simulink model "Rebuild"  (R2024b)
settings: Solver=VariableStepAuto  StartTime=0.0  StopTime=12  RelTol=1e-3
values from neighbouring files (symbols this model uses):
  A = 1.1    [RT14e_Parameters.m]    (also in RT15e_Parameters.m = 1.088; RT15evo_Parameters.m = 1.088)
  Aero_balance = 55    [RT14e_Parameters.m]    (also in RT15e_Parameters.m; RT15evo_Parameters.m)
  Aeromaps_ON = 0    [SIM_setup.m]
  air_density = 1.2    [SIM_setup.m]
  Balance_FW = Data_FW_STD(1:end,2)    [RT15e_Parameters.m]    (also in RT15evo_Parameters.m)
  Balance_R_11 = Data_R_11(1:end,2)    [RT15e_Parameters.m]    (also in RT15evo_Parameters.m)
  Br_coef_of_friction_F = 0.33    [RT14e_Parameters.m]    (also in RT15e_Parameters.m; RT15evo_Parameters.m)
  Br_coef_of_friction_R = 0.33    [RT14e_Parameters.m]    (also in RT15e_Parameters.m; RT15evo_Parameters.m)
  Br_pistons_area_F = 3617.26/1e6    (= 0.00361726)    [RT14e_Parameters.m]    (also in RT15e_Parameters.m; RT15evo_Parameters.m)
  Br_pistons_area_R = 2026.83/1e6    (= 0.00202683)    [RT14e_Parameters.m]    (also in RT15e_Parameters.m; RT15evo_Parameters.m)
  CdA = 1.31*A    (= 1.441)    [RT14e_Parameters.m]    (also in RT15e_Parameters.m = 1.700544; RT15evo_Parameters.m = 1.700544)
  CdA_FW = Data_FW_STD(1:end,3)    [RT15e_Parameters.m]    (also in RT15evo_Parameters.m)
  CdA_R_11 = Data_R_11(1:end,3)    [RT15e_Parameters.m]    (also in RT15evo_Parameters.m)
  ClA = 3.3*A    (= 3.63)    [RT14e_Parameters.m]    (also in RT15e_Parameters.m = 4.36288; RT15evo_Parameters.m = 4.36288)
  ClA_FW = Data_FW_STD(1:end,4)    [RT15e_Parameters.m]    (also in RT15evo_Parameters.m)
  ClA_R_11 = Data_R_11(1:end,4)    [RT15e_Parameters.m]    (also in RT15evo_Parameters.m)
  CoG_z = 0.35    [RT14e_Parameters.m]    (also in RT15e_Parameters.m = 0.28495; RT15evo_Parameters.m = 0.28495)
  Default_Fz_FL = Default_Fz_F/2 + (Default_Fz_F*CoG_y/Track_Front)    [RT14e_Parameters.m]    (also in RT15e_Parameters.m; RT15evo_Parameters.m)
  Default_Fz_FR = Default_Fz_F/2 - (Default_Fz_F*CoG_y/Track_Front)    [RT14e_Parameters.m]    (also in RT15e_Parameters.m; RT15evo_Parameters.m)
  Default_Fz_RL = Default_Fz_R/2 + (Default_Fz_R*CoG_y/Track_Rear)    [RT14e_Parameters.m]    (also in RT15e_Parameters.m; RT15evo_Parameters.m)
  Default_Fz_RR = Default_Fz_R/2 - (Default_Fz_R*CoG_y/Track_Rear)    [RT14e_Parameters.m]    (also in RT15e_Parameters.m; RT15evo_Parameters.m)
  Effective_br_disk_r_F = 0.0905    [RT14e_Parameters.m]    (also in RT15e_Parameters.m; RT15evo_Parameters.m)
  Effective_br_disk_r_R = 0.0895    [RT14e_Parameters.m]    (also in RT15e_Parameters.m; RT15evo_Parameters.m)
  Front_brake_balance = 0.0    (= 0)    [RT14e_Parameters.m]    (also in RT15e_Parameters.m; RT15evo_Parameters.m)
  Front_brake_pump_area = 153.94    [RT14e_Parameters.m]    (also in RT15e_Parameters.m; RT15evo_Parameters.m)
  Front_desired_brake_p_balance = 0.6    [RT14e_Parameters.m]    (also in RT15e_Parameters.m; RT15evo_Parameters.m)
  FW_Setup = Data_FW_STD(1:end,1)    [RT15e_Parameters.m]    (also in RT15evo_Parameters.m)
  Fx = Data_Fx(2:end,3:end)    [RT14e_Parameters.m]    (also in RT15e_Parameters.m; RT15evo_Parameters.m)
  Fy = Data_Fy(2:end,3:end)    [RT14e_Parameters.m]    (also in RT15e_Parameters.m; RT15evo_Parameters.m)
  Fz = Data_Fy(2:end,2)    [RT14e_Parameters.m]    (also in RT15e_Parameters.m; RT15evo_Parameters.m)
  g = 9.81    [SIM_setup.m]
  Gear_ratio = 12.9    [RT14e_Parameters.m]    (also in RT15e_Parameters.m; RT15evo_Parameters.m)
  Iz_wehicle = 120    [RT14e_Parameters.m]    (also in RT15e_Parameters.m; RT15evo_Parameters.m)
  Iz_wheel = 0.15    [RT14e_Parameters.m]    (also in RT15e_Parameters.m; RT15evo_Parameters.m)
  Lf = Wheelbase - CoG_x    (= 0.77)    [RT14e_Parameters.m]    (also in RT15e_Parameters.m = 0.7504; RT15evo_Parameters.m = 0.7504)
  LLTD = 0.45    [RT14e_Parameters.m]    (also in RT15e_Parameters.m = 0.55; RT15evo_Parameters.m = 0.55)
  Lock_brake_balance = false    [RT14e_Parameters.m]    (also in RT15e_Parameters.m; RT15evo_Parameters.m)
  Lr = Wheelbase - Lf    (= 0.755)    [RT14e_Parameters.m]    (also in RT15e_Parameters.m = 0.7746; RT15evo_Parameters.m = 0.7746)
  Mass = Vehicle_mass + Driver_mass    (= 290)    [RT14e_Parameters.m]    (also in RT15e_Parameters.m = 265; RT15evo_Parameters.m)
  Motor_maximum_power = 35366    [RT14e_Parameters.m]    (also in RT15e_Parameters.m; RT15evo_Parameters.m)
  RB_torque_setting_1 = -2    [RT14e_Parameters.m]    (also in RT15e_Parameters.m; RT15evo_Parameters.m)
  RB_torque_setting_10 = -20    [RT14e_Parameters.m]    (also in RT15e_Parameters.m; RT15evo_Parameters.m)
  RB_torque_setting_2 = -4    [RT14e_Parameters.m]    (also in RT15e_Parameters.m; RT15evo_Parameters.m)
  RB_torque_setting_3 = -6    [RT14e_Parameters.m]    (also in RT15e_Parameters.m; RT15evo_Parameters.m)
  RB_torque_setting_4 = -8    [RT14e_Parameters.m]    (also in RT15e_Parameters.m; RT15evo_Parameters.m)
  RB_torque_setting_5 = -10    [RT14e_Parameters.m]    (also in RT15e_Parameters.m; RT15evo_Parameters.m)
  RB_torque_setting_6 = -12    [RT14e_Parameters.m]    (also in RT15e_Parameters.m; RT15evo_Parameters.m)
  RB_torque_setting_7 = -14    [RT14e_Parameters.m]    (also in RT15e_Parameters.m; RT15evo_Parameters.m)
  RB_torque_setting_8 = -16    [RT14e_Parameters.m]    (also in RT15e_Parameters.m; RT15evo_Parameters.m)
  RB_torque_setting_9 = -18    [RT14e_Parameters.m]    (also in RT15e_Parameters.m; RT15evo_Parameters.m)
  Rear_brake_pump_area = 198.56    [RT14e_Parameters.m]    (also in RT15e_Parameters.m; RT15evo_Parameters.m)
  Roll_Angle_11 = Data_R_11(1:end,1)    [RT15e_Parameters.m]    (also in RT15evo_Parameters.m)
  SA = Data_Fy(1,3:end)    [RT14e_Parameters.m]    (also in RT15e_Parameters.m; RT15evo_Parameters.m)
  SR = Data_Fx(1,3:end)    [RT14e_Parameters.m]    (also in RT15e_Parameters.m; RT15evo_Parameters.m)
  start_acc_x = double(start_acc_x_ts.Data)    [SIM_setup.m]
  start_acc_y = double(start_acc_y_ts.Data)    [SIM_setup.m]
  start_time = 1188    [SIM_setup.m]
  start_velocity_x = double(start_velocity_x_ts.Data)    [SIM_setup.m]
  start_velocity_y = double(start_velocity_y_ts.Data)    [SIM_setup.m]
  start_yaw_acc = double(start_yaw_acc_ts.Data)    [SIM_setup.m]
  start_yaw_rate = double(start_yaw_rate_ts.Data)    [SIM_setup.m]
  Static_Camber_FL = 0    [RT14e_Parameters.m]    (also in RT15e_Parameters.m; RT15evo_Parameters.m)
  Static_Camber_FR = 0    [RT14e_Parameters.m]    (also in RT15e_Parameters.m; RT15evo_Parameters.m)
  Static_Camber_RL = 0    [RT14e_Parameters.m]    (also in RT15e_Parameters.m; RT15evo_Parameters.m)
  Static_Camber_RR = 0    [RT14e_Parameters.m]    (also in RT15e_Parameters.m; RT15evo_Parameters.m)
  Static_Toe_FL = 0    [RT14e_Parameters.m]    (also in RT15e_Parameters.m; RT15evo_Parameters.m)
  Static_Toe_FR = 0    [RT14e_Parameters.m]    (also in RT15e_Parameters.m; RT15evo_Parameters.m)
  Static_Toe_RL = 0    [RT14e_Parameters.m]    (also in RT15e_Parameters.m; RT15evo_Parameters.m)
  Static_Toe_RR = 0    [RT14e_Parameters.m]    (also in RT15e_Parameters.m; RT15evo_Parameters.m)
  Steering_Angle_FL = Data_Steering(1:end,2)    [RT14e_Parameters.m]    (also in RT15e_Parameters.m; RT15evo_Parameters.m)
  Steering_Angle_FR = Data_Steering(1:end,3)    [RT14e_Parameters.m]    (also in RT15e_Parameters.m; RT15evo_Parameters.m)
  Steering_Wheel_Angle = Data_Steering(1:end,1)    [RT14e_Parameters.m]    (also in RT15e_Parameters.m; RT15evo_Parameters.m)
  Tire_radius = 0.203    [RT14e_Parameters.m]    (also in RT15e_Parameters.m; RT15evo_Parameters.m)
  Torque_limit_2 = Motor_maximum_torque*0.2    (= 5.82)    [RT14e_Parameters.m]    (also in RT15e_Parameters.m; RT15evo_Parameters.m)
  Torque_limit_3 = Motor_maximum_torque*0.3    (= 8.73)    [RT14e_Parameters.m]    (also in RT15e_Parameters.m; RT15evo_Parameters.m)
  Torque_limit_4 = Motor_maximum_torque*0.4    (= 11.64)    [RT14e_Parameters.m]    (also in RT15e_Parameters.m; RT15evo_Parameters.m)
  Torque_limit_5 = Motor_maximum_torque*0.5    (= 14.55)    [RT14e_Parameters.m]    (also in RT15e_Parameters.m; RT15evo_Parameters.m)
  Torque_limit_6 = Motor_maximum_torque*0.6    (= 17.46)    [RT14e_Parameters.m]    (also in RT15e_Parameters.m; RT15evo_Parameters.m)
  Torque_limit_7 = Motor_maximum_torque*0.7    (= 20.37)    [RT14e_Parameters.m]    (also in RT15e_Parameters.m; RT15evo_Parameters.m)
  Torque_limit_8 = Motor_maximum_torque*0.8    (= 23.28)    [RT14e_Parameters.m]    (also in RT15e_Parameters.m; RT15evo_Parameters.m)
  Torque_limit_9 = 29.1    [RT14e_Parameters.m]    (also in RT15e_Parameters.m; RT15evo_Parameters.m)
  Torque_limit_max = Motor_maximum_torque    (= 29.1)    [RT14e_Parameters.m]    (also in RT15e_Parameters.m; RT15evo_Parameters.m)
  Torque_limit_min = Motor_maximum_torque*0.1    (= 2.91)    [RT14e_Parameters.m]    (also in RT15e_Parameters.m; RT15evo_Parameters.m)
  Torque_limit_set = 10    [RT14e_Parameters.m]    (also in RT15e_Parameters.m; RT15evo_Parameters.m)
  Track_Front = 1.2    [RT14e_Parameters.m]    (also in RT15e_Parameters.m; RT15evo_Parameters.m)
  Track_Rear = 1.18    [RT14e_Parameters.m]    (also in RT15e_Parameters.m; RT15evo_Parameters.m)
  TV_ON = 0    [SIM_setup.m]
  TV_RB_understeer_gradient_1 = -0.5    [RT14e_Parameters.m]    (also in RT15e_Parameters.m; RT15evo_Parameters.m)
  TV_RB_understeer_gradient_10 = 0.005    [RT14e_Parameters.m]    (also in RT15e_Parameters.m; RT15evo_Parameters.m)
  TV_RB_understeer_gradient_2 = -0.1    [RT14e_Parameters.m]    (also in RT15e_Parameters.m; RT15evo_Parameters.m)
  TV_RB_understeer_gradient_3 = 0.08    [RT14e_Parameters.m]    (also in RT15e_Parameters.m; RT15evo_Parameters.m)
  TV_RB_understeer_gradient_4 = 0.06    [RT14e_Parameters.m]    (also in RT15e_Parameters.m; RT15evo_Parameters.m)
  TV_RB_understeer_gradient_5 = 0.05    [RT14e_Parameters.m]    (also in RT15e_Parameters.m; RT15evo_Parameters.m)
  TV_RB_understeer_gradient_6 = 0.04    [RT14e_Parameters.m]    (also in RT15e_Parameters.m; RT15evo_Parameters.m)
  TV_RB_understeer_gradient_7 = 0.03    [RT14e_Parameters.m]    (also in RT15e_Parameters.m; RT15evo_Parameters.m)
  TV_RB_understeer_gradient_8 = 0.02    [RT14e_Parameters.m]    (also in RT15e_Parameters.m; RT15evo_Parameters.m)
  TV_RB_understeer_gradient_9 = 0.01    [RT14e_Parameters.m]    (also in RT15e_Parameters.m; RT15evo_Parameters.m)
  TV_understeer_gradient_1 = -0.5    [RT14e_Parameters.m]    (also in RT15e_Parameters.m; RT15evo_Parameters.m)
  TV_understeer_gradient_10 = 0.002    [RT14e_Parameters.m]    (also in RT15e_Parameters.m; RT15evo_Parameters.m)
  TV_understeer_gradient_2 = -0.1    [RT14e_Parameters.m]    (also in RT15e_Parameters.m; RT15evo_Parameters.m)
  TV_understeer_gradient_3 = 0.06    [RT14e_Parameters.m]    (also in RT15e_Parameters.m; RT15evo_Parameters.m)
  TV_understeer_gradient_4 = 0.05    [RT14e_Parameters.m]    (also in RT15e_Parameters.m; RT15evo_Parameters.m)
  TV_understeer_gradient_5 = 0.04    [RT14e_Parameters.m]    (also in RT15e_Parameters.m; RT15evo_Parameters.m)
  TV_understeer_gradient_6 = 0.03    [RT14e_Parameters.m]    (also in RT15e_Parameters.m; RT15evo_Parameters.m)
  TV_understeer_gradient_7 = 0.02    [RT14e_Parameters.m]    (also in RT15e_Parameters.m; RT15evo_Parameters.m)
  TV_understeer_gradient_8 = 0.01    [RT14e_Parameters.m]    (also in RT15e_Parameters.m; RT15evo_Parameters.m)
  TV_understeer_gradient_9 = 0.005    [RT14e_Parameters.m]    (also in RT15e_Parameters.m; RT15evo_Parameters.m)
  Vx_APPS_ON = 1    [SIM_setup.m]
  Wheel_rolling_resistance = 0.055    [RT14e_Parameters.m]    (also in RT15e_Parameters.m; RT15evo_Parameters.m)
  Wheelbase = 1.525    [RT14e_Parameters.m]    (also in RT15e_Parameters.m; RT15evo_Parameters.m)
undefined symbols (not defined in the file or in its folder): Actual_Torque_Value_RL, Actual_Torque_Value_RR, aero_balance, APPS, Brake_Pressure_Front, Brake_Pressure_Rear, Cl, lateral_load_transfer_distribution, maths_GPS_Velocity, Max_Torque, rad, s, Steering_position, tire_radius, wheel_base, Wheel_Speed_RL, Wheel_Speed_RR, Xsens_MTI_670_accX, Xsens_MTI_670_accY, Xsens_MTI_670_gyrZ
libraries: simulink x30, simulink_extras x11, slpidlib x9, dspstat3 x4, slrealtimeloglib x1, aerolibconvert2 x1
(part 6 of 6)

== system Rebuild/Main/Powertrain/Motors/Control Algorithms/TV Algorithm/Torque Vectoring/Subsystem1/Switch Case Action Subsystem3 ==
  Torque After TV RL [Nm] not saturated : Inport
  Torque After TV RR [Nm] not saturated : Inport  Port=2
  Action Port : ActionPort
  Bus Creator : BusCreator  Inputs=2
  Saturation : Saturate  UpperLimit=0  LowerLimit=RB_torque_setting_4
  Saturation1 : Saturate  UpperLimit=0  LowerLimit=RB_torque_setting_4
  Out1 : Outport
  wires:
  Torque After TV RL [Nm] not saturated/1 -> Saturation/1
  Bus Creator/1 -> Out1/1
  Saturation/1 -> Bus Creator/1  "Torque After TV RL [Nm]"
  Torque After TV RR [Nm] not saturated/1 -> Saturation1/1
  Saturation1/1 -> Bus Creator/2  "Torque After TV RR [Nm]"

== system Rebuild/Main/Powertrain/Motors/Control Algorithms/TV Algorithm/Torque Vectoring/Subsystem1/Switch Case Action Subsystem4 ==
  Torque After TV RL [Nm] not saturated : Inport
  Torque After TV RR [Nm] not saturated : Inport  Port=2
  Action Port : ActionPort
  Bus Creator : BusCreator  Inputs=2
  Saturation : Saturate  UpperLimit=0  LowerLimit=RB_torque_setting_5
  Saturation1 : Saturate  UpperLimit=0  LowerLimit=RB_torque_setting_5
  Out1 : Outport
  wires:
  Torque After TV RL [Nm] not saturated/1 -> Saturation/1
  Bus Creator/1 -> Out1/1
  Saturation/1 -> Bus Creator/1  "Torque After TV RL [Nm]"
  Torque After TV RR [Nm] not saturated/1 -> Saturation1/1
  Saturation1/1 -> Bus Creator/2  "Torque After TV RR [Nm]"

== system Rebuild/Main/Powertrain/Motors/Control Algorithms/TV Algorithm/Torque Vectoring/Subsystem1/Switch Case Action Subsystem5 ==
  Torque After TV RL [Nm] not saturated : Inport
  Torque After TV RR [Nm] not saturated : Inport  Port=2
  Action Port : ActionPort
  Bus Creator : BusCreator  Inputs=2
  Saturation : Saturate  UpperLimit=0  LowerLimit=RB_torque_setting_6
  Saturation1 : Saturate  UpperLimit=0  LowerLimit=RB_torque_setting_6
  Out1 : Outport
  wires:
  Torque After TV RL [Nm] not saturated/1 -> Saturation/1
  Bus Creator/1 -> Out1/1
  Saturation/1 -> Bus Creator/1  "Torque After TV RL [Nm]"
  Torque After TV RR [Nm] not saturated/1 -> Saturation1/1
  Saturation1/1 -> Bus Creator/2  "Torque After TV RR [Nm]"

== system Rebuild/Main/Powertrain/Motors/Control Algorithms/TV Algorithm/Torque Vectoring/Subsystem1/Switch Case Action Subsystem6 ==
  Torque After TV RL [Nm] not saturated : Inport
  Torque After TV RR [Nm] not saturated : Inport  Port=2
  Action Port : ActionPort
  Bus Creator : BusCreator  Inputs=2
  Saturation : Saturate  UpperLimit=0  LowerLimit=RB_torque_setting_7
  Saturation1 : Saturate  UpperLimit=0  LowerLimit=RB_torque_setting_7
  Out1 : Outport
  wires:
  Torque After TV RL [Nm] not saturated/1 -> Saturation/1
  Bus Creator/1 -> Out1/1
  Saturation/1 -> Bus Creator/1  "Torque After TV RL [Nm]"
  Torque After TV RR [Nm] not saturated/1 -> Saturation1/1
  Saturation1/1 -> Bus Creator/2  "Torque After TV RR [Nm]"

== system Rebuild/Main/Powertrain/Motors/Control Algorithms/TV Algorithm/Torque Vectoring/Subsystem1/Switch Case Action Subsystem7 ==
  Torque After TV RL [Nm] not saturated : Inport
  Torque After TV RR [Nm] not saturated : Inport  Port=2
  Action Port : ActionPort
  Bus Creator : BusCreator  Inputs=2
  Saturation : Saturate  UpperLimit=0  LowerLimit=RB_torque_setting_8
  Saturation1 : Saturate  UpperLimit=0  LowerLimit=RB_torque_setting_8
  Out1 : Outport
  wires:
  Torque After TV RL [Nm] not saturated/1 -> Saturation/1
  Bus Creator/1 -> Out1/1
  Saturation/1 -> Bus Creator/1  "Torque After TV RL [Nm]"
  Torque After TV RR [Nm] not saturated/1 -> Saturation1/1
  Saturation1/1 -> Bus Creator/2  "Torque After TV RR [Nm]"

== system Rebuild/Main/Powertrain/Motors/Control Algorithms/TV Algorithm/Torque Vectoring/Subsystem1/Switch Case Action Subsystem8 ==
  Torque After TV RL [Nm] not saturated : Inport
  Torque After TV RR [Nm] not saturated : Inport  Port=2
  Action Port : ActionPort
  Bus Creator : BusCreator  Inputs=2
  Saturation : Saturate  UpperLimit=0  LowerLimit=RB_torque_setting_9
  Saturation1 : Saturate  UpperLimit=0  LowerLimit=RB_torque_setting_9
  Out1 : Outport
  wires:
  Torque After TV RL [Nm] not saturated/1 -> Saturation/1
  Bus Creator/1 -> Out1/1
  Saturation/1 -> Bus Creator/1  "Torque After TV RL [Nm]"
  Torque After TV RR [Nm] not saturated/1 -> Saturation1/1
  Saturation1/1 -> Bus Creator/2  "Torque After TV RR [Nm]"

== system Rebuild/Main/Powertrain/Motors/Control Algorithms/TV Algorithm/Torque Vectoring/Subsystem1/Switch Case Action Subsystem9 ==
  Torque After TV RL [Nm] not saturated : Inport
  Torque After TV RR [Nm] not saturated : Inport  Port=2
  Action Port : ActionPort
  Bus Creator : BusCreator  Inputs=2
  Saturation : Saturate  UpperLimit=0  LowerLimit=RB_torque_setting_10
  Saturation1 : Saturate  UpperLimit=0  LowerLimit=RB_torque_setting_10
  Out1 : Outport
  wires:
  Torque After TV RL [Nm] not saturated/1 -> Saturation/1
  Bus Creator/1 -> Out1/1
  Saturation/1 -> Bus Creator/1  "Torque After TV RL [Nm]"
  Torque After TV RR [Nm] not saturated/1 -> Saturation1/1
  Saturation1/1 -> Bus Creator/2  "Torque After TV RR [Nm]"

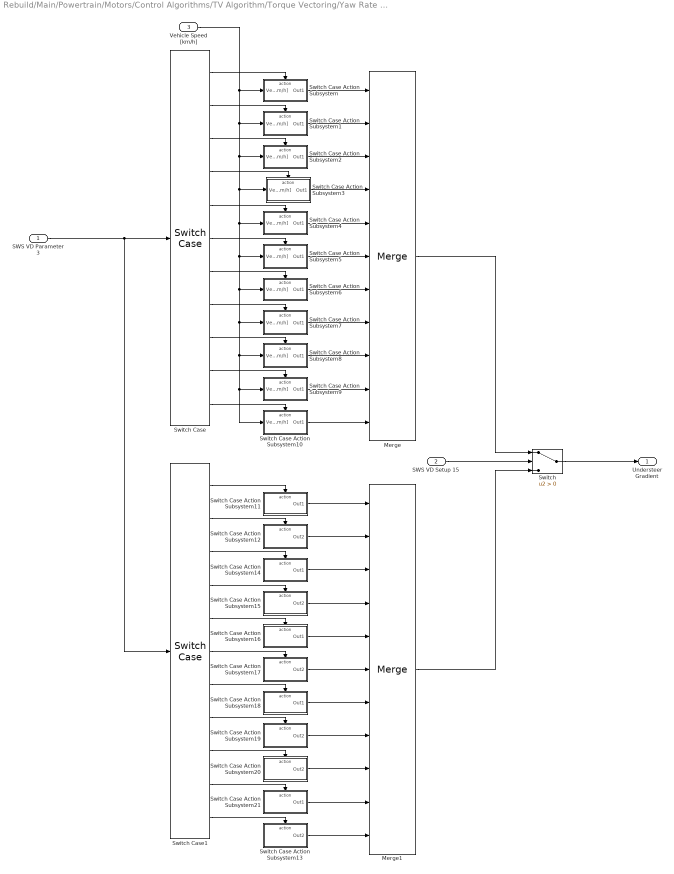
== system Rebuild/Main/Powertrain/Motors/Control Algorithms/TV Algorithm/Torque Vectoring/Yaw Rate Calculation/Understeer Gradeint Selection ==
  SWS VD Parameter 3 : Inport
  SWS VD Setup 15 : Inport  Port=2
  Vehicle Speed [km/h] : Inport  Port=3
  Merge : Merge  Inputs=11
  Merge1 : Merge  Inputs=11
  Switch : Switch  Criteria=u2 > Threshold  SaturateOnIntegerOverflow=off  InputSameDT=off
  Switch Case : SwitchCase  CaseConditions={1,2,3,4,5,6,7,8,9,10}
  Switch Case Action Subsystem : Subsystem  TreatAsAtomicUnit=on
  Switch Case Action Subsystem1 : Subsystem  TreatAsAtomicUnit=on
  Switch Case Action Subsystem10 : Subsystem  TreatAsAtomicUnit=on
  Switch Case Action Subsystem11 : Subsystem  TreatAsAtomicUnit=on
  Switch Case Action Subsystem12 : Subsystem  TreatAsAtomicUnit=on
  Switch Case Action Subsystem13 : Subsystem  TreatAsAtomicUnit=on
  Switch Case Action Subsystem14 : Subsystem  TreatAsAtomicUnit=on
  Switch Case Action Subsystem15 : Subsystem  TreatAsAtomicUnit=on
  Switch Case Action Subsystem16 : Subsystem  TreatAsAtomicUnit=on
  Switch Case Action Subsystem17 : Subsystem  TreatAsAtomicUnit=on
  Switch Case Action Subsystem18 : Subsystem  TreatAsAtomicUnit=on
  Switch Case Action Subsystem19 : Subsystem  TreatAsAtomicUnit=on
  Switch Case Action Subsystem2 : Subsystem  TreatAsAtomicUnit=on
  Switch Case Action Subsystem20 : Subsystem  TreatAsAtomicUnit=on
  Switch Case Action Subsystem21 : Subsystem  TreatAsAtomicUnit=on
  Switch Case Action Subsystem3 : Subsystem  TreatAsAtomicUnit=on
  Switch Case Action Subsystem4 : Subsystem  TreatAsAtomicUnit=on
  Switch Case Action Subsystem5 : Subsystem  TreatAsAtomicUnit=on
  Switch Case Action Subsystem6 : Subsystem  TreatAsAtomicUnit=on
  Switch Case Action Subsystem7 : Subsystem  TreatAsAtomicUnit=on
  Switch Case Action Subsystem8 : Subsystem  TreatAsAtomicUnit=on
  Switch Case Action Subsystem9 : Subsystem  TreatAsAtomicUnit=on
  Switch Case1 : SwitchCase  CaseConditions={1,2,3,4,5,6,7,8,9,10}
  Understeer Gradient : Outport
  wires:
  Switch Case Action Subsystem1/1(Out1) -> Merge/2
  Switch Case Action Subsystem5/1(Out1) -> Merge/6
  Switch Case/7 -> Switch Case Action Subsystem6/Action
  Switch Case Action Subsystem2/1(Out1) -> Merge/3
  Switch Case/1 -> Switch Case Action Subsystem/Action
  Switch Case Action Subsystem/1(Out1) -> Merge/1
  Switch Case/6 -> Switch Case Action Subsystem5/Action
  Switch Case/4 -> Switch Case Action Subsystem3/Action
  Switch Case/3 -> Switch Case Action Subsystem2/Action
  Switch Case/5 -> Switch Case Action Subsystem4/Action
  Switch Case Action Subsystem10/1(Out1) -> Merge/11
  Switch Case Action Subsystem3/1(Out1) -> Merge/4
  Switch Case Action Subsystem7/1(Out1) -> Merge/8
  Switch Case Action Subsystem6/1(Out1) -> Merge/7
  Switch Case/8 -> Switch Case Action Subsystem7/Action
  Switch Case Action Subsystem9/1(Out1) -> Merge/10
  Switch Case Action Subsystem4/1(Out1) -> Merge/5
  Switch Case Action Subsystem8/1(Out1) -> Merge/9
  Switch Case/2 -> Switch Case Action Subsystem1/Action
  Switch Case/10 -> Switch Case Action Subsystem9/Action
  Switch Case/9 -> Switch Case Action Subsystem8/Action
  Switch Case/11 -> Switch Case Action Subsystem10/Action
  SWS VD Parameter 3/1 -> Switch Case1/1, Switch Case/1
  Switch Case1/11 -> Switch Case Action Subsystem13/Action
  Switch Case1/9 -> Switch Case Action Subsystem20/Action
  Switch Case1/10 -> Switch Case Action Subsystem21/Action
  Switch Case1/2 -> Switch Case Action Subsystem12/Action
  Switch Case Action Subsystem20/1(Out2) -> Merge1/9
  Switch Case Action Subsystem16/1(Out1) -> Merge1/5
  Switch Case Action Subsystem21/1(Out1) -> Merge1/10
  Switch Case1/8 -> Switch Case Action Subsystem19/Action
  Switch Case Action Subsystem18/1(Out1) -> Merge1/7
  Merge1/1 -> Switch/3
  Switch Case Action Subsystem19/1(Out2) -> Merge1/8
  Switch Case Action Subsystem15/1(Out2) -> Merge1/4
  Switch Case Action Subsystem13/1(Out2) -> Merge1/11
  Switch Case1/5 -> Switch Case Action Subsystem16/Action
  Switch Case1/3 -> Switch Case Action Subsystem14/Action
  Switch Case1/4 -> Switch Case Action Subsystem15/Action
  Switch Case1/6 -> Switch Case Action Subsystem17/Action
  Switch Case Action Subsystem11/1(Out1) -> Merge1/1
  Switch Case1/1 -> Switch Case Action Subsystem11/Action
  Switch Case Action Subsystem14/1(Out1) -> Merge1/3
  Switch Case1/7 -> Switch Case Action Subsystem18/Action
  Switch Case Action Subsystem17/1(Out2) -> Merge1/6
  Switch Case Action Subsystem12/1(Out2) -> Merge1/2
  SWS VD Setup 15/1 -> Switch/2
  Merge/1 -> Switch/1
  Switch/1 -> Understeer Gradient/1
  Vehicle Speed [km/h]/1 -> Switch Case Action Subsystem/1(Vehicle Speed [km/h]), Switch Case Action Subsystem1/1(Vehicle Speed [km/h]), Switch Case Action Subsystem2/1(Vehicle Speed [km/h]), Switch Case Action Subsystem3/1(Vehicle Speed [km/h]), Switch Case Action Subsystem4/1(Vehicle Speed [km/h]), Switch Case Action Subsystem5/1(Vehicle Speed [km/h]), Switch Case Action Subsystem6/1(Vehicle Speed [km/h]), Switch Case Action Subsystem7/1(Vehicle Speed [km/h]), Switch Case Action Subsystem8/1(Vehicle Speed [km/h]), Switch Case Action Subsystem10/1(Vehicle Speed [km/h]), Switch Case Action Subsystem9/1(Vehicle Speed [km/h])

== system Rebuild/Main/Powertrain/Motors/Control Algorithms/TV Algorithm/Torque Vectoring/RB Yaw Rate Calculation/Understeer Gradeint Selection/Switch Case Action Subsystem11 ==
  Action Port : ActionPort
  Constant1 : Constant  Value=TV_RB_understeer_gradient_1
  Out1 : Outport
  wires:
  Constant1/1 -> Out1/1

== system Rebuild/Main/Powertrain/Motors/Control Algorithms/TV Algorithm/Torque Vectoring/RB Yaw Rate Calculation/Understeer Gradeint Selection/Switch Case Action Subsystem12 ==
  Action Port : ActionPort
  Constant : Constant  Value=TV_RB_understeer_gradient_2
  Out2 : Outport
  wires:
  Constant/1 -> Out2/1

== system Rebuild/Main/Powertrain/Motors/Control Algorithms/TV Algorithm/Torque Vectoring/RB Yaw Rate Calculation/Understeer Gradeint Selection/Switch Case Action Subsystem13 ==
  Action Port : ActionPort
  Constant : Constant  Value=TV_RB_understeer_gradient_6
  Out2 : Outport
  wires:
  Constant/1 -> Out2/1

== system Rebuild/Main/Powertrain/Motors/Control Algorithms/TV Algorithm/Torque Vectoring/RB Yaw Rate Calculation/Understeer Gradeint Selection/Switch Case Action Subsystem14 ==
  Action Port : ActionPort
  Constant1 : Constant  Value=TV_RB_understeer_gradient_3
  Out1 : Outport
  wires:
  Constant1/1 -> Out1/1

== system Rebuild/Main/Powertrain/Motors/Control Algorithms/TV Algorithm/Torque Vectoring/RB Yaw Rate Calculation/Understeer Gradeint Selection/Switch Case Action Subsystem15 ==
  Action Port : ActionPort
  Constant : Constant  Value=TV_RB_understeer_gradient_4
  Out2 : Outport
  wires:
  Constant/1 -> Out2/1

== system Rebuild/Main/Powertrain/Motors/Control Algorithms/TV Algorithm/Torque Vectoring/RB Yaw Rate Calculation/Understeer Gradeint Selection/Switch Case Action Subsystem16 ==
  Action Port : ActionPort
  Constant : Constant  Value=TV_RB_understeer_gradient_5
  Out1 : Outport
  wires:
  Constant/1 -> Out1/1

== system Rebuild/Main/Powertrain/Motors/Control Algorithms/TV Algorithm/Torque Vectoring/RB Yaw Rate Calculation/Understeer Gradeint Selection/Switch Case Action Subsystem17 ==
  Action Port : ActionPort
  Constant : Constant  Value=TV_RB_understeer_gradient_6
  Out2 : Outport
  wires:
  Constant/1 -> Out2/1

== system Rebuild/Main/Powertrain/Motors/Control Algorithms/TV Algorithm/Torque Vectoring/RB Yaw Rate Calculation/Understeer Gradeint Selection/Switch Case Action Subsystem18 ==
  Action Port : ActionPort
  Constant : Constant  Value=TV_RB_understeer_gradient_7
  Out1 : Outport
  wires:
  Constant/1 -> Out1/1

== system Rebuild/Main/Powertrain/Motors/Control Algorithms/TV Algorithm/Torque Vectoring/RB Yaw Rate Calculation/Understeer Gradeint Selection/Switch Case Action Subsystem19 ==
  Action Port : ActionPort
  Constant : Constant  Value=TV_RB_understeer_gradient_8
  Out2 : Outport
  wires:
  Constant/1 -> Out2/1

== system Rebuild/Main/Powertrain/Motors/Control Algorithms/TV Algorithm/Torque Vectoring/RB Yaw Rate Calculation/Understeer Gradeint Selection/Switch Case Action Subsystem20 ==
  Action Port : ActionPort
  Constant : Constant  Value=TV_RB_understeer_gradient_9
  Out2 : Outport
  wires:
  Constant/1 -> Out2/1

== system Rebuild/Main/Powertrain/Motors/Control Algorithms/TV Algorithm/Torque Vectoring/RB Yaw Rate Calculation/Understeer Gradeint Selection/Switch Case Action Subsystem21 ==
  Action Port : ActionPort
  Constant : Constant  Value=TV_RB_understeer_gradient_10
  Out1 : Outport
  wires:
  Constant/1 -> Out1/1

== system Rebuild/Main/Powertrain/Motors/Control Algorithms/TV Algorithm/Torque Vectoring/Yaw Rate Calculation/Understeer Gradeint Selection/Switch Case Action Subsystem ==
  Vehicle Speed [km/h] : Inport
  Action Port : ActionPort
  1-D Lookup Table : Lookup_n-D  NumberOfTableDimensions=1  BreakpointsForDimension1=[25;30;35;40;45;50;55;60;65;70;75;80]  Table=[0.03;0.06;0.08;0.1;0.12;0.15;0.22;0.3;0.35;0.42;0.48;0.55]  InternalRulePriority=Speed  RndMeth=Simplest
  Saturation : Saturate  UpperLimit=80  LowerLimit=25
  Saturation1 : Saturate  UpperLimit=0.55  LowerLimit=0.03
  Out1 : Outport
  wires:
  1-D Lookup Table/1 -> Saturation1/1
  Saturation1/1 -> Out1/1
  Vehicle Speed [km/h]/1 -> Saturation/1
  Saturation/1 -> 1-D Lookup Table/1

== system Rebuild/Main/Powertrain/Motors/Control Algorithms/TV Algorithm/Torque Vectoring/Yaw Rate Calculation/Understeer Gradeint Selection/Switch Case Action Subsystem1 ==
  Vehicle Speed [km/h] : Inport
  Action Port : ActionPort
  1-D Lookup Table : Lookup_n-D  NumberOfTableDimensions=1  BreakpointsForDimension1=[25;30;35;40;45;50;55;60;65;70;75;80]  Table=[0.02;0.04;0.06;0.08;0.1;0.14;0.16;0.2;0.25;0.32;0.38;0.45]  InternalRulePriority=Speed  RndMeth=Simplest
  Saturation : Saturate  UpperLimit=80  LowerLimit=25
  Saturation1 : Saturate  UpperLimit=0.45  LowerLimit=0.02
  Out1 : Outport
  wires:
  Vehicle Speed [km/h]/1 -> Saturation/1
  Saturation/1 -> 1-D Lookup Table/1
  1-D Lookup Table/1 -> Saturation1/1
  Saturation1/1 -> Out1/1

== system Rebuild/Main/Powertrain/Motors/Control Algorithms/TV Algorithm/Torque Vectoring/Yaw Rate Calculation/Understeer Gradeint Selection/Switch Case Action Subsystem10 ==
  Vehicle Speed [km/h] : Inport
  Action Port : ActionPort
  1-D Lookup Table : Lookup_n-D  NumberOfTableDimensions=1  BreakpointsForDimension1=[25;30;35;40;45;50;55;60;65;70;75;80]  Table=[0.003;0.005;0.008;0.01;0.03;0.05;0.08;0.12;0.15;0.18;0.25;0.3]  InternalRulePriority=Speed  RndMeth=Simplest
  Saturation : Saturate  UpperLimit=80  LowerLimit=25
  Saturation1 : Saturate  UpperLimit=0.3  LowerLimit=0.001
  Out1 : Outport
  wires:
  1-D Lookup Table/1 -> Saturation1/1
  Vehicle Speed [km/h]/1 -> Saturation/1
  Saturation1/1 -> Out1/1
  Saturation/1 -> 1-D Lookup Table/1

== system Rebuild/Main/Powertrain/Motors/Control Algorithms/TV Algorithm/Torque Vectoring/Yaw Rate Calculation/Understeer Gradeint Selection/Switch Case Action Subsystem11 ==
  Action Port : ActionPort
  Constant1 : Constant  Value=TV_understeer_gradient_1
  Out1 : Outport
  wires:
  Constant1/1 -> Out1/1

== system Rebuild/Main/Powertrain/Motors/Control Algorithms/TV Algorithm/Torque Vectoring/Yaw Rate Calculation/Understeer Gradeint Selection/Switch Case Action Subsystem12 ==
  Action Port : ActionPort
  Constant : Constant  Value=TV_understeer_gradient_2
  Out2 : Outport
  wires:
  Constant/1 -> Out2/1

== system Rebuild/Main/Powertrain/Motors/Control Algorithms/TV Algorithm/Torque Vectoring/Yaw Rate Calculation/Understeer Gradeint Selection/Switch Case Action Subsystem13 ==
  Action Port : ActionPort
  Constant : Constant  Value=TV_understeer_gradient_8
  Out2 : Outport
  wires:
  Constant/1 -> Out2/1

== system Rebuild/Main/Powertrain/Motors/Control Algorithms/TV Algorithm/Torque Vectoring/Yaw Rate Calculation/Understeer Gradeint Selection/Switch Case Action Subsystem14 ==
  Action Port : ActionPort
  Constant1 : Constant  Value=TV_understeer_gradient_3
  Out1 : Outport
  wires:
  Constant1/1 -> Out1/1

== system Rebuild/Main/Powertrain/Motors/Control Algorithms/TV Algorithm/Torque Vectoring/Yaw Rate Calculation/Understeer Gradeint Selection/Switch Case Action Subsystem15 ==
  Action Port : ActionPort
  Constant : Constant  Value=TV_understeer_gradient_4
  Out2 : Outport
  wires:
  Constant/1 -> Out2/1

== system Rebuild/Main/Powertrain/Motors/Control Algorithms/TV Algorithm/Torque Vectoring/Yaw Rate Calculation/Understeer Gradeint Selection/Switch Case Action Subsystem16 ==
  Action Port : ActionPort
  Constant : Constant  Value=TV_understeer_gradient_5
  Out1 : Outport
  wires:
  Constant/1 -> Out1/1

== system Rebuild/Main/Powertrain/Motors/Control Algorithms/TV Algorithm/Torque Vectoring/Yaw Rate Calculation/Understeer Gradeint Selection/Switch Case Action Subsystem17 ==
  Action Port : ActionPort
  Constant : Constant  Value=TV_understeer_gradient_6
  Out2 : Outport
  wires:
  Constant/1 -> Out2/1

== system Rebuild/Main/Powertrain/Motors/Control Algorithms/TV Algorithm/Torque Vectoring/Yaw Rate Calculation/Understeer Gradeint Selection/Switch Case Action Subsystem18 ==
  Action Port : ActionPort
  Constant : Constant  Value=TV_understeer_gradient_7
  Out1 : Outport
  wires:
  Constant/1 -> Out1/1

== system Rebuild/Main/Powertrain/Motors/Control Algorithms/TV Algorithm/Torque Vectoring/Yaw Rate Calculation/Understeer Gradeint Selection/Switch Case Action Subsystem19 ==
  Action Port : ActionPort
  Constant : Constant  Value=TV_understeer_gradient_8
  Out2 : Outport
  wires:
  Constant/1 -> Out2/1

== system Rebuild/Main/Powertrain/Motors/Control Algorithms/TV Algorithm/Torque Vectoring/Yaw Rate Calculation/Understeer Gradeint Selection/Switch Case Action Subsystem2 ==
  Vehicle Speed [km/h] : Inport
  Action Port : ActionPort
  1-D Lookup Table1 : Lookup_n-D  NumberOfTableDimensions=1  BreakpointsForDimension1=[25;30;35;40;45;50;55;60;65;70;75;80]  Table=[0.01;0.02;0.04;0.06;0.08;0.12;0.16;0.22;0.28;0.35;0.42;0.5]  InternalRulePriority=Speed  RndMeth=Simplest
  Saturation2 : Saturate  UpperLimit=80  LowerLimit=25
  Saturation3 : Saturate  LowerLimit=0.01
  Out1 : Outport
  wires:
  Vehicle Speed [km/h]/1 -> Saturation2/1
  Saturation3/1 -> Out1/1
  Saturation2/1 -> 1-D Lookup Table1/1
  1-D Lookup Table1/1 -> Saturation3/1

== system Rebuild/Main/Powertrain/Motors/Control Algorithms/TV Algorithm/Torque Vectoring/Yaw Rate Calculation/Understeer Gradeint Selection/Switch Case Action Subsystem20 ==
  Action Port : ActionPort
  Constant : Constant  Value=TV_understeer_gradient_9
  Out2 : Outport
  wires:
  Constant/1 -> Out2/1

== system Rebuild/Main/Powertrain/Motors/Control Algorithms/TV Algorithm/Torque Vectoring/Yaw Rate Calculation/Understeer Gradeint Selection/Switch Case Action Subsystem21 ==
  Action Port : ActionPort
  Constant : Constant  Value=TV_understeer_gradient_10
  Out1 : Outport
  wires:
  Constant/1 -> Out1/1

== system Rebuild/Main/Powertrain/Motors/Control Algorithms/TV Algorithm/Torque Vectoring/Yaw Rate Calculation/Understeer Gradeint Selection/Switch Case Action Subsystem3 ==
  Vehicle Speed [km/h] : Inport
  Action Port : ActionPort
  1-D Lookup Table : Lookup_n-D  NumberOfTableDimensions=1  BreakpointsForDimension1=[25;30;35;40;45;50;55;60;65;70;75;80]  Table=[0.005;0.02;0.04;0.06;0.08;0.1;0.12;0.15;0.18;0.25;0.32;0.4]  InternalRulePriority=Speed  RndMeth=Simplest
  Saturation : Saturate  UpperLimit=80  LowerLimit=25
  Saturation1 : Saturate  UpperLimit=0.4  LowerLimit=0.005
  Out1 : Outport
  wires:
  Vehicle Speed [km/h]/1 -> Saturation/1
  Saturation1/1 -> Out1/1
  1-D Lookup Table/1 -> Saturation1/1
  Saturation/1 -> 1-D Lookup Table/1

== system Rebuild/Main/Powertrain/Motors/Control Algorithms/TV Algorithm/Torque Vectoring/Yaw Rate Calculation/Understeer Gradeint Selection/Switch Case Action Subsystem4 ==
  Vehicle Speed [km/h] : Inport
  Action Port : ActionPort
  1-D Lookup Table : Lookup_n-D  NumberOfTableDimensions=1  BreakpointsForDimension1=[25;30;35;40;45;50;55;60;65;70;75;80]  Table=[0.003;0.006;0.01;0.03;0.06;0.08;0.1;0.13;0.16;0.2;0.28;0.35]  InternalRulePriority=Speed  RndMeth=Simplest
  Saturation : Saturate  UpperLimit=80  LowerLimit=25
  Saturation1 : Saturate  UpperLimit=0.35  LowerLimit=0.003
  Out1 : Outport
  wires:
  1-D Lookup Table/1 -> Saturation1/1
  Vehicle Speed [km/h]/1 -> Saturation/1
  Saturation1/1 -> Out1/1
  Saturation/1 -> 1-D Lookup Table/1

== system Rebuild/Main/Powertrain/Motors/Control Algorithms/TV Algorithm/Torque Vectoring/Yaw Rate Calculation/Understeer Gradeint Selection/Switch Case Action Subsystem5 ==
  Vehicle Speed [km/h] : Inport
  Action Port : ActionPort
  1-D Lookup Table : Lookup_n-D  NumberOfTableDimensions=1  BreakpointsForDimension1=[25;30;35;40;45;50;55;60;65;70;75;80]  Table=[0.003;0.005;0.008;0.01;0.03;0.05;0.08;0.12;0.15;0.18;0.25;0.3]  InternalRulePriority=Speed  RndMeth=Simplest
  Saturation : Saturate  UpperLimit=80  LowerLimit=25
  Saturation1 : Saturate  UpperLimit=0.3  LowerLimit=0.003
  Out1 : Outport
  wires:
  Saturation/1 -> 1-D Lookup Table/1
  Saturation1/1 -> Out1/1
  1-D Lookup Table/1 -> Saturation1/1
  Vehicle Speed [km/h]/1 -> Saturation/1

== system Rebuild/Main/Powertrain/Motors/Control Algorithms/TV Algorithm/Torque Vectoring/Yaw Rate Calculation/Understeer Gradeint Selection/Switch Case Action Subsystem6 ==
  Vehicle Speed [km/h] : Inport
  Action Port : ActionPort
  1-D Lookup Table : Lookup_n-D  NumberOfTableDimensions=1  BreakpointsForDimension1=[25;30;35;40;45;50;55;60;65;70;75;80]  Table=[0.002;0.003;0.005;0.008;0.01;0.03;0.06;0.09;0.12;0.16;0.2;0.25]  InternalRulePriority=Speed  RndMeth=Simplest
  Saturation : Saturate  UpperLimit=80  LowerLimit=25
  Saturation1 : Saturate  UpperLimit=0.25  LowerLimit=0.002
  Out1 : Outport
  wires:
  Vehicle Speed [km/h]/1 -> Saturation/1
  Saturation1/1 -> Out1/1
  Saturation/1 -> 1-D Lookup Table/1
  1-D Lookup Table/1 -> Saturation1/1

== system Rebuild/Main/Powertrain/Motors/Control Algorithms/TV Algorithm/Torque Vectoring/Yaw Rate Calculation/Understeer Gradeint Selection/Switch Case Action Subsystem7 ==
  Vehicle Speed [km/h] : Inport
  Action Port : ActionPort
  1-D Lookup Table : Lookup_n-D  NumberOfTableDimensions=1  BreakpointsForDimension1=[25;30;35;40;45;50;55;60;65;70;75;80]  Table=[0.001;0.002;0.005;0.007;0.008;0.015;0.03;0.06;0.08;0.12;0.15;0.2]  InternalRulePriority=Speed  RndMeth=Simplest
  Saturation : Saturate  UpperLimit=80  LowerLimit=25
  Saturation1 : Saturate  UpperLimit=0.2  LowerLimit=0.001
  Out1 : Outport
  wires:
  Saturation1/1 -> Out1/1
  1-D Lookup Table/1 -> Saturation1/1
  Saturation/1 -> 1-D Lookup Table/1
  Vehicle Speed [km/h]/1 -> Saturation/1

== system Rebuild/Main/Powertrain/Motors/Control Algorithms/TV Algorithm/Torque Vectoring/Yaw Rate Calculation/Understeer Gradeint Selection/Switch Case Action Subsystem8 ==
  Vehicle Speed [km/h] : Inport
  Action Port : ActionPort
  1-D Lookup Table : Lookup_n-D  NumberOfTableDimensions=1  BreakpointsForDimension1=[25;30;35;40;45;50;55;60;65;70;75;80]  Table=[0.001;0.002;0.005;0.007;0.008;0.009;0.01;0.02;0.03;0.04;0.07;0.1]  InternalRulePriority=Speed  RndMeth=Simplest
  Saturation : Saturate  UpperLimit=80  LowerLimit=25
  Saturation1 : Saturate  UpperLimit=0.12  LowerLimit=0.001
  Out1 : Outport
  wires:
  Vehicle Speed [km/h]/1 -> Saturation/1
  Saturation1/1 -> Out1/1
  Saturation/1 -> 1-D Lookup Table/1
  1-D Lookup Table/1 -> Saturation1/1

== system Rebuild/Main/Powertrain/Motors/Control Algorithms/TV Algorithm/Torque Vectoring/Yaw Rate Calculation/Understeer Gradeint Selection/Switch Case Action Subsystem9 ==
  Vehicle Speed [km/h] : Inport
  Action Port : ActionPort
  1-D Lookup Table1 : Lookup_n-D  NumberOfTableDimensions=1  BreakpointsForDimension1=[25;30;35;40;45;50;55;60;65;70;75;80]  Table=[0.001;0.003;0.007;0.009;0.01;0.013;0.018;0.022;0.03;0.04;0.07;0.1]  InternalRulePriority=Speed  RndMeth=Simplest
  Saturation : Saturate  UpperLimit=80  LowerLimit=25
  Saturation2 : Saturate  UpperLimit=0.1  LowerLimit=0.001
  Out1 : Outport
  wires:
  Vehicle Speed [km/h]/1 -> Saturation/1
  Saturation/1 -> 1-D Lookup Table1/1
  Saturation2/1 -> Out1/1
  1-D Lookup Table1/1 -> Saturation2/1
